simulink model "RocketBooster_P1"  (R2024b)
settings: Solver=VariableStepAuto  StartTime=0.0  StopTime=20  RelTol=1e-3
undefined symbols (not defined in the file): A, alpha0, B, C, D, dFT_test, Fw_test, x0
settings Model: Creator=maria  LastModifiedBy=maria

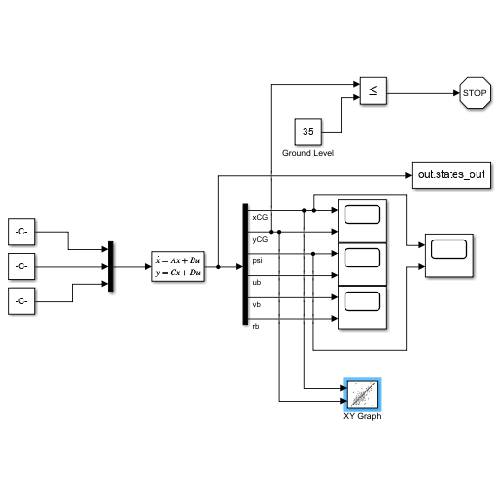
[thumbnail: Simulink's stored preview of the top-level diagram]
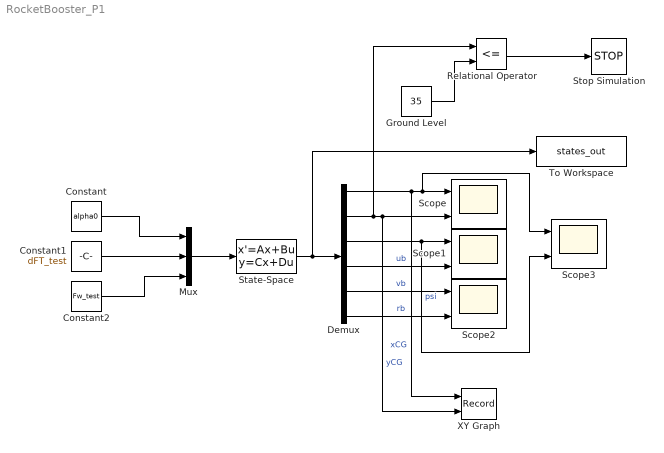
== system RocketBooster_P1 ==
  Constant : Constant  Value=alpha0
  Constant1 : Constant  Value=dFT_test
  Constant2 : Constant  Value=Fw_test
  Demux : Demux  Outputs=6
  Ground Level : Constant  Value=35
  Mux : Mux  Inputs=3
  Relational Operator : RelationalOperator  Operator=<=  OutDataTypeStr=boolean  RndMeth=Simplest  InputSameDT=off
  Scope{,1..3} (4 alike) : Scope  NumInputPorts=2
  State-Space : StateSpace  A=A  B=B  C=C  D=D  InitialCondition=x0
  Stop Simulation : Stop
  To Workspace : ToWorkspace  VariableName=states_out  SaveFormat=Structure With Time  SampleTime=-1
  XY Graph : Record  FileSettingsInternal="{\"entries\":[{\"content\":{\"excelSettings\":{\"content\":{},\"type\":\"Streamout.ExcelSettings\"}},\"type\":\"Streamout.FileSettingStorage\",\"uuid\":\"\"}],\"packageUris\":[\"http:\\/\\/schema.mathworks.com\\/mf0\\/streamout_blocks\\/R2020a\"],\"version\":\"1.0\"}"  Layout=[1 1]  SignalsInternal="{\"entries\":[{\"content\":{\"signals\":[{\"content\":{\"blockPath\":[],\"dimensions\":[1],\"domain\":\"\",\"lineColor\":\"#a2142f\",\"plots\":[ 1 ],\"port\":1,\"sid\":[\"\"],\"signalID\":1,\"signalName\":\"xCG\"},\"type\":\"RecordBlkView.Signal\",\"uuid\":\"\"},{\"content\":{\"blockPath\":[],\"dimensions\":[1],\"domain\":\"\",\"lineColor\":\"#139fff\",\"plots\":[ 1 ],\"port\":2,\"sid\":[\"\"],\"signalID\":2,\"signalName\":\"yCG\"},\"type\":\"RecordBlkView.Signal\",\"uuid\":\"\"}]},\"type\":\"RecordBlkView.InputSignals\",\"uuid\":\"\"}],\"packageUris\":[\"http:\\/\\/schema.mathworks.com\\/mf0\\/streamout_blocks\\/R2020a\"],\"version\":\"1.0\"}"  VisualizationBindings="{\"xyplotplugin\":{\"info\":[{\"series\":[{\"bindingParametersList\":[{\"parameter\":\"X-Axis\",\"signalID\":1,\"signalName\":\"xCG\"},{\"parameter\":\"Y-Axis\",\"signalID\":2,\"signalName\":\"yCG\"}],\"seriesID\":0}],\"subplotID\":1}]}}"  CompatibilityTag=XY
  wires:
  Constant1/1 -> Mux/2
  Constant/1 -> Mux/1
  Mux/1 -> State-Space/1
  Demux/6 -> Scope2/2  "rb"
  Demux/5 -> Scope2/1  "vb"
  Demux/4 -> Scope1/2  "ub"
  Demux/3 -> Scope3/2, Scope1/1  "psi"
  Demux/2 -> XY Graph/2, Scope/2, Relational Operator/1  "yCG"
  Demux/1 -> XY Graph/1, Scope3/1, Scope/1  "xCG"
  State-Space/1 -> To Workspace/1, Demux/1
  Relational Operator/1 -> Stop Simulation/1
  Constant2/1 -> Mux/3
  Ground Level/1 -> Relational Operator/2
